simulink model "w1p1"  (R2020a)
settings: Solver=VariableStepAuto  StartTime=0.0  StopTime=10  MaxStep=0.001  RelTol=1e-3
model workspace (MAT data in the model file):
  B1 = Simulink.Parameter
  B1.Value = 50
  B1.DataType = 'auto'
  B1.Dimensions = [1 1]
  K1 = Simulink.Parameter
  K1.Value = 50
  K1.DataType = 'auto'
  K1.Dimensions = [1 1]
  K12 = Simulink.Parameter
  K12.Value = 50
  K12.DataType = 'auto'
  K12.Dimensions = [1 1]
  M1 = Simulink.Parameter
  M1.Value = 100
  M1.DataType = 'auto'
  M1.Dimensions = [1 1]
  M2 = Simulink.Parameter
  M2.Value = 120
  M2.DataType = 'auto'
  M2.Dimensions = [1 1]
settings Model: Creator=avn19  LastModifiedBy=avn19

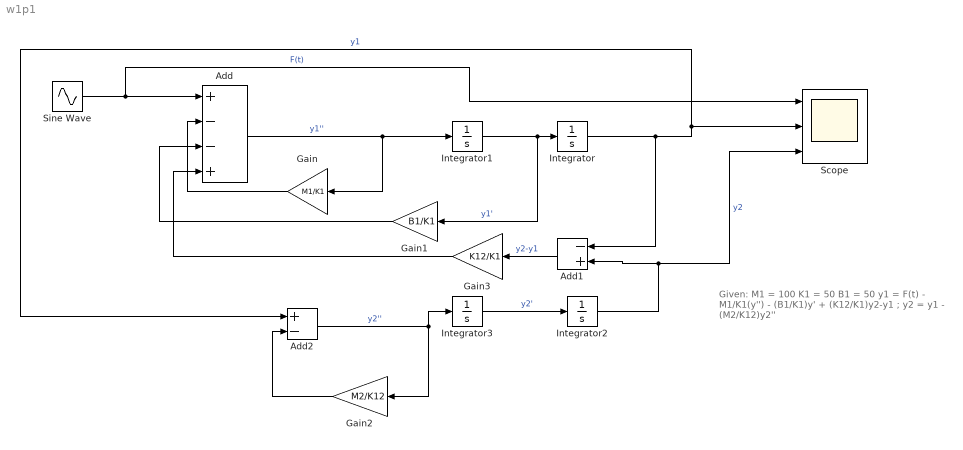
== system w1p1 ==
  note: Given:
      | M1 = 100
      | K1 = 50
      | B1 = 50
      |
      | y1 = F(t) - M1/K1(y'') - (B1/K1)y' + (K12/K1)y2-y1 ;
      | y2 = y1 - (M2/K12)y2''
  Add : Sum  Inputs=+--+
  Add1 : Sum  Inputs=-+
  Add2 : Sum  Inputs=+-
  Gain : Gain  Gain=M1/K1
  Gain1 : Gain  Gain=B1/K1
  Gain2 : Gain  Gain=M2/K12
  Gain3 : Gain  Gain=K12/K1
  Integrator{,1..3} (4 alike) : Integrator
  Scope : Scope  NumInputPorts=3
  Sine Wave : Sin  Amplitude=2  Frequency=10*2*pi  SampleTime=0
  wires:
  Integrator/1 -> Add1/1, Add2/1, Scope/2  "y1"
  Integrator1/1 -> Gain1/1, Integrator/1  "y1'"
  Add/1 -> Gain/1, Integrator1/1  "y1''"
  Gain/1 -> Add/2
  Gain1/1 -> Add/3
  Sine Wave/1 -> Add/1, Scope/1  "F(t)"
  Integrator2/1 -> Add1/2, Scope/3  "y2"
  Integrator3/1 -> Integrator2/1  "y2'"
  Add2/1 -> Integrator3/1, Gain2/1  "y2''"
  Gain2/1 -> Add2/2
  Add1/1 -> Gain3/1  "y2-y1"
  Gain3/1 -> Add/4
